simulink model "MotoreCC"  (R2017a)
settings: Solver=VariableStepAuto  StartTime=0.0  StopTime=10.0  RelTol=1e-3
values from neighbouring files (symbols this model uses):
  b = 0.1    [MotoreCC.m]
  J = 0.01    [MotoreCC.m]
  K = 0.01    [MotoreCC.m]
  L = 0.5    [MotoreCC.m]
  R = 1    [MotoreCC.m]
settings Model: Creator=Michele  LastModifiedBy=Michele

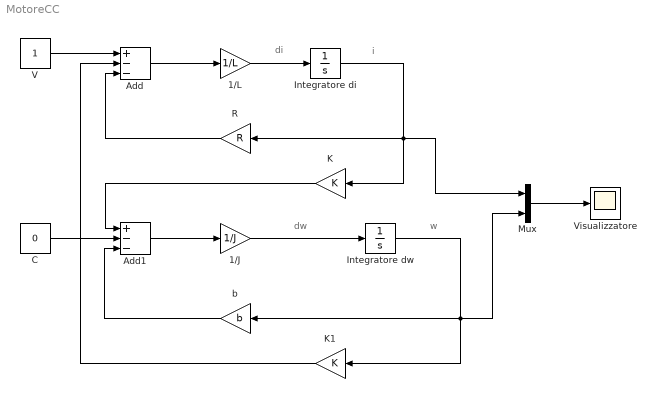
== system MotoreCC ==
  note: w
  note: dw
  note: i
  note: di
  1/J : Gain  Gain=1/J
  1/L : Gain  Gain=1/L
  Add : Sum  Inputs=+--
  Add1 : Sum  Inputs=+--
  C : Constant  Value=0
  Integratore di : Integrator
  Integratore dw : Integrator
  K : Gain  Gain=K
  K1 : Gain  Gain=K
  Mux : Mux  Inputs=2
  R : Gain  Gain=R
  V : Constant
  Visualizzatore : Scope
  b : Gain  Gain=b
  wires:
  V/1 -> Add/1
  C/1 -> Add1/2
  Add/1 -> 1/L/1
  Add1/1 -> 1/J/1
  1/L/1 -> Integratore di/1
  1/J/1 -> Integratore dw/1
  Integratore di/1 -> Mux/1, K/1, R/1
  Integratore dw/1 -> Mux/2, K1/1, b/1
  R/1 -> Add/3
  K/1 -> Add1/1
  K1/1 -> Add/2
  b/1 -> Add1/3
  Mux/1 -> Visualizzatore/1
